simulink model "competenciaparches"  (R2020a)
settings: Solver=VariableStepAuto  StartTime=0.0  StopTime=10.0  RelTol=1e-3
undefined symbols (not defined in the file): c1, c2, m1, m2, P10, P20
settings Model: Creator=curie  LastModifiedBy=curie

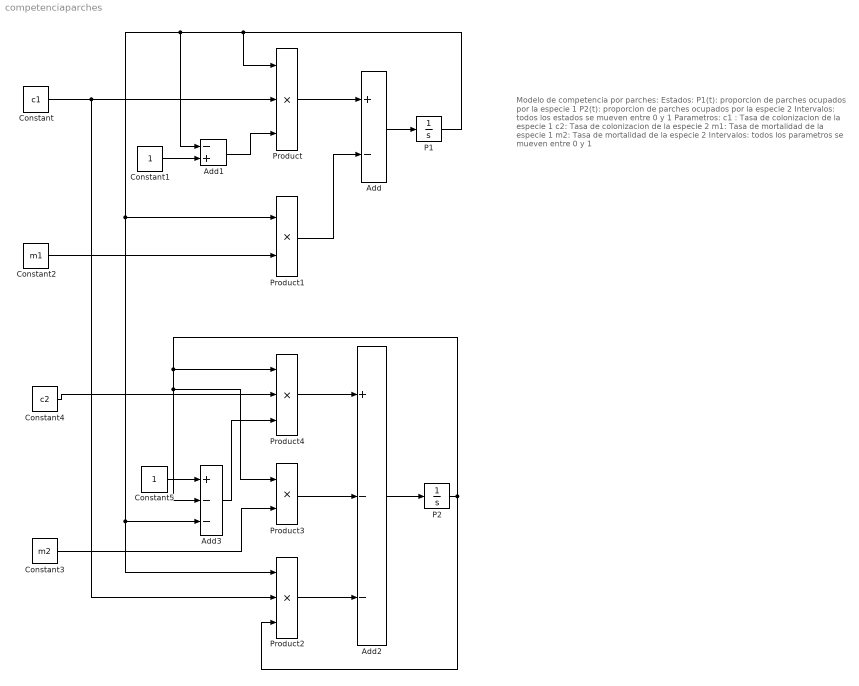
== system competenciaparches ==
  note: Modelo de competencia por parches:
      |
      | Estados:
      | P1(t): proporcion de parches ocupados por la especie 1
      | P2(t): proporcion de parches ocupados por la especie 2
      |
      | Intervalos: todos los estados se mueven entre 0 y 1
      |
      | Parametros:
      | c1 : Tasa de colonizacion de la especie 1
      | c2: Tasa de colonizacion de la especie 2
      | m1: Tasa de mortalidad de la especie 1
      | m2: Tasa de mortalidad de la especie 2
      |
      | Intervalos: todos los parametros se mueven entre 0 y 1
  Add : Sum  Inputs=+-
  Add1 : Sum  Inputs=-+
  Add2 : Sum  Inputs=+--
  Add3 : Sum  Inputs=+--
  Constant : Constant  Value=c1
  Constant1 : Constant
  Constant2 : Constant  Value=m1
  Constant3 : Constant  Value=m2
  Constant4 : Constant  Value=c2
  Constant5 : Constant
  P1 : Integrator  InitialCondition=P10
  P2 : Integrator  InitialCondition=P20
  Product : Product  Inputs=3
  Product1 : Product
  Product2 : Product  Inputs=3
  Product3 : Product
  Product4 : Product  Inputs=3
  wires:
  P1/1 -> Product/1, Add1/1, Product2/1, Add3/3, Product1/1
  Constant/1 -> Product2/2, Product/2
  Add/1 -> P1/1
  Product/1 -> Add/1
  Add1/1 -> Product/3
  Constant1/1 -> Add1/2
  Product1/1 -> Add/2
  Constant2/1 -> Product1/2
  Add2/1 -> P2/1
  Product2/1 -> Add2/3
  Product3/1 -> Add2/2
  Product4/1 -> Add2/1
  P2/1 -> Product2/3, Product3/1, Add3/2, Product4/1
  Constant4/1 -> Product4/2
  Add3/1 -> Product4/3
  Constant5/1 -> Add3/1
  Constant3/1 -> Product3/2
